simulink model "VCU_GearMgnt"  (R2023b)
settings: Solver=FixedStepDiscrete  StartTime=0.0  StopTime=10  FixedStep=0.01  RelTol=1e-3
undefined symbols (not defined in the file or in its folder): MOTOR_RPM_EN_GEAR, VEH_SPEED_EN_GEAR
libraries: simulink x24
settings Model: Creator=Administrator  LastModifiedBy=Administrator
settings OptimizationCC: DefaultParameterBehavior=Inlined  EnhancedBackFolding=on  PassReuseOutputArgsAs=Individual arguments  ZeroExternalMemoryAtStartup=off  ZeroInternalMemoryAtStartup=off  OptimizeBlockOrder=speed  DifferentSizesBufferReuse=on  OptimizationCustomize=off  EfficientTunableParamExpr=on
settings DebuggingCC: ParameterTunabilityLossMsg=error
settings HardwareCC: ProdBitPerPointer=32  ProdBitPerSizeT=32  ProdBitPerPtrDiffT=32  ProdLargestAtomicInteger=Long  ProdLargestAtomicFloat=Double  ProdWordSize=32  ProdHWDeviceType=ARM Compatible->ARM Cortex-M
settings SFSimCC: MATLABDynamicMemAlloc=off
settings RTWCC: Description=Embedded Coder  SystemTargetFile=ert.tlc  GenCodeOnly=on  TemplateMakefile=ert_default_tmf  GenerateReport=on  IncludeHyperlinkInReport=on  LaunchReport=on  GenerateTraceInfo=on  GenerateTraceReport=on  GenerateCodeReplacementReport=on
settings CodeAppCC: ForceParamTrailComments=on  IgnoreCustomStorageClasses=off  OperatorAnnotations=on  SimulinkDataObjDesc=on  SFDataObjDesc=on  InsertBlockDesc=on
settings ERTTargetCC: TargetLangStandard=C99 (ISO)  GenerateSampleERTMain=on  InlinedParameterPlacement=NonHierarchical  ERTCustomFileTemplate=example_file_process.tlc

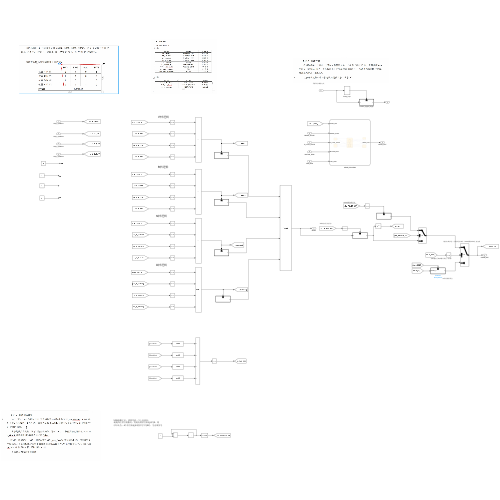
[thumbnail: Simulink's stored preview of the top-level diagram]
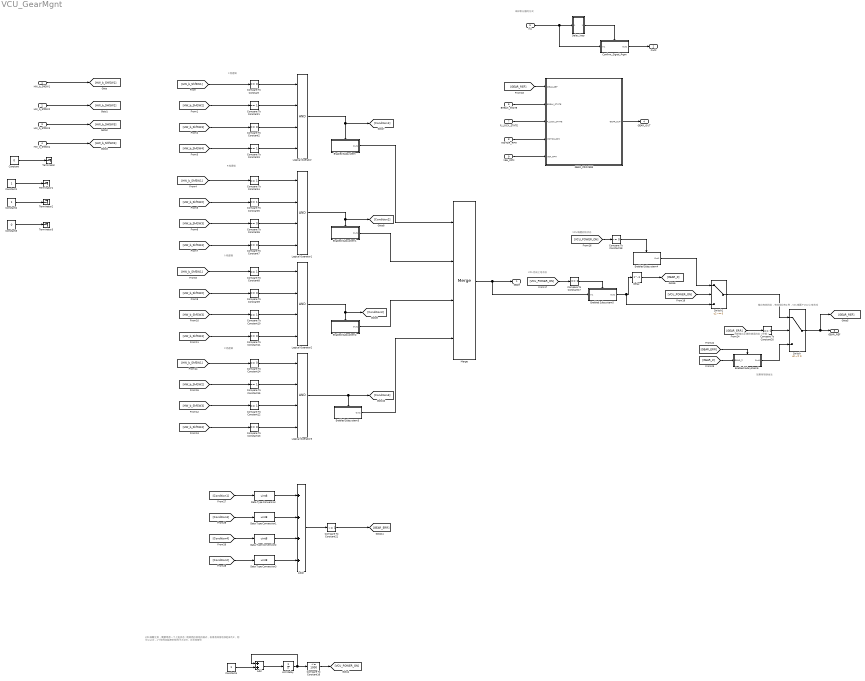
== system VCU_GearMgnt ==
  note: P档逻辑
  note: 输出有效挡位，有效挡位有2种，VCU唤醒+VCU上电完成
  note: 如果有错误发生
  note: VCU唤醒初始状态
  note: VCU唤醒之后，需要考虑一个上电状态;
      | 观测挡位信号的格式，发现有效信号加起来为2，则
      | 可以认为，4个信号加起来的信号不为2时，为无效信号
  note: 采样积分器的方式
  note: VCU完成上电状态
  note: 判断输出正确和错误挡位（仲裁）
  note: R档逻辑
  note: N档逻辑
  note: D档逻辑
  HW_b_ShfSW1 : Inport
  HW_b_ShfSW2 : Inport  Port=2
  HW_b_ShfSW3 : Inport  Port=3
  HW_b_ShfSW4 : Inport  Port=4
  In1 : Inport  Port=5
  BREAK_STATE : Inport  Port=6
  P_LOCK_STATE : Inport  Port=7
  MOTOR_RPM : Inport  Port=8
  VEH_RPM : Inport  Port=9
  Add : Sum
  Add2 : Sum  Inputs=++++
  Compare To Constant{,2,6..7,9,11,13..14,17,20} (10 alike) : simulink/Logic and Bit Operations/Compare To Constant  relop===  const=0  OutDataTypeStr=boolean
  Compare To Constant{1,3..5,8,10,12,15} (8 alike) : simulink/Logic and Bit Operations/Compare To Constant  relop===  const=1  OutDataTypeStr=boolean
  Compare To Constant16 : simulink/Logic and Bit Operations/Compare To Constant  relop=<=  const=1000  OutDataTypeStr=boolean
  Compare To Constant18 : simulink/Logic and Bit Operations/Compare To Constant  relop=~=  const=0  OutDataTypeStr=boolean
  Compare To Constant21 : simulink/Logic and Bit Operations/Compare To Constant  relop=~=  const=1  OutDataTypeStr=boolean
  Confirm_Signal_Prgm : Subsystem  TreatAsAtomicUnit=on
  Constant : Constant  Value=0
  Constant1 : Constant
  Constant2 : Constant
  Constant3 : Constant  Value=0
  Constant4 : Constant
  Data Type Conversion{,1..3} (4 alike) : DataTypeConversion  OutDataTypeStr=uint8  SaturateOnIntegerOverflow=off  RndMeth=Floor
  Delay : Delay  DelayLength=1  InputProcessing=Columns as channels (frame based)
  Delay_loop : Subsystem
  Enabled Subsystem : Subsystem  TreatAsAtomicUnit=on
  Enabled Subsystem1 : Subsystem  TreatAsAtomicUnit=on
  Enabled Subsystem2 : Subsystem  TreatAsAtomicUnit=on
  Enabled Subsystem3 : Subsystem  TreatAsAtomicUnit=on
  Enabled Subsystem4 : Subsystem  TreatAsAtomicUnit=on
  Enabled Subsystem5 : Subsystem  TreatAsAtomicUnit=on
  Enabled Subsystem6 : Subsystem  TreatAsAtomicUnit=on
  GEAR_PROCESS : Stateflow chart  TreatAsAtomicUnit=on
  Logical Operator{,1..3} (4 alike) : Logic  Inputs=4  AllPortsSameDT=off  OutDataTypeStr=boolean
  Merge : Merge  Inputs=4
  Switch : Switch  Criteria=u2 ~= 0  SaturateOnIntegerOverflow=off  InputSameDT=off
  Switch1 : Switch  Criteria=u2 ~= 0  SaturateOnIntegerOverflow=off  InputSameDT=off
  Terminator{,1..3} (4 alike) : Terminator
  Unit Delay : UnitDelay  SampleTime=-1  HasFrameUpgradeWarning=on
  GEAR : Outport
  Out2 : Outport  Port=2
  GEAR_REF : Outport  Port=3
  GEAR_OUT : Outport  Port=4
  wires:
  [HW_b_ShfSW1] -> Compare To Constant/1
  [HW_b_ShfSW2] -> Compare To Constant1/1
  [HW_b_ShfSW3] -> Compare To Constant2/1
  [HW_b_ShfSW4] -> Compare To Constant3/1
  Compare To Constant/1 -> Logical Operator/1
  Compare To Constant1/1 -> Logical Operator/2
  Compare To Constant2/1 -> Logical Operator/3
  Compare To Constant3/1 -> Logical Operator/4
  Compare To Constant7/1 -> Logical Operator1/4
  Compare To Constant6/1 -> Logical Operator1/3
  Compare To Constant5/1 -> Logical Operator1/2
  Compare To Constant4/1 -> Logical Operator1/1
  [HW_b_ShfSW4] -> Compare To Constant7/1
  [HW_b_ShfSW3] -> Compare To Constant6/1
  [HW_b_ShfSW2] -> Compare To Constant5/1
  [HW_b_ShfSW1] -> Compare To Constant4/1
  [HW_b_ShfSW1] -> Compare To Constant8/1
  [HW_b_ShfSW2] -> Compare To Constant9/1
  [HW_b_ShfSW3] -> Compare To Constant10/1
  [HW_b_ShfSW4] -> Compare To Constant11/1
  Compare To Constant8/1 -> Logical Operator2/1
  Compare To Constant9/1 -> Logical Operator2/2
  Compare To Constant10/1 -> Logical Operator2/3
  Compare To Constant11/1 -> Logical Operator2/4
  Compare To Constant13/1 -> Logical Operator3/4
  Compare To Constant12/1 -> Logical Operator3/3
  Compare To Constant15/1 -> Logical Operator3/2
  Compare To Constant14/1 -> Logical Operator3/1
  [HW_b_ShfSW4] -> Compare To Constant13/1
  [HW_b_ShfSW3] -> Compare To Constant12/1
  [HW_b_ShfSW2] -> Compare To Constant15/1
  [HW_b_ShfSW1] -> Compare To Constant14/1
  Logical Operator/1 -> [Condition1], Enabled Subsystem/Enable
  Logical Operator1/1 -> Enabled Subsystem1/Enable, [Condition2]
  Logical Operator2/1 -> [Condition3], Enabled Subsystem2/Enable
  Logical Operator3/1 -> Enabled Subsystem3/Enable, [Condition4]
  Enabled Subsystem/1(Out1) -> Merge/1
  Enabled Subsystem1/1(Out1) -> Merge/2
  Enabled Subsystem2/1(Out1) -> Merge/3
  Enabled Subsystem3/1(Out1) -> Merge/4
  Merge/1 -> Enabled Subsystem5/1(In1), GEAR/1
  HW_b_ShfSW1/1 -> [HW_b_ShfSW1]
  HW_b_ShfSW2/1 -> [HW_b_ShfSW2]
  HW_b_ShfSW3/1 -> [HW_b_ShfSW3]
  HW_b_ShfSW4/1 -> [HW_b_ShfSW4]
  Constant/1 -> Terminator/1
  Constant1/1 -> Terminator1/1
  Constant2/1 -> Terminator2/1
  Constant3/1 -> Terminator3/1
  In1/1 -> Confirm_Signal_Prgm/1(In1), Delay_loop/1(In1)
  Delay_loop/1(Out2) -> Confirm_Signal_Prgm/Enable
  Confirm_Signal_Prgm/1(Out1) -> Out2/1
  Constant4/1 -> Add/2
  Add/1 -> Unit Delay/1
  Unit Delay/1 -> Add/1, Compare To Constant16/1
  Compare To Constant16/1 -> [VCU_POWER_ON]
  [VCU_POWER_ON] -> Compare To Constant18/1
  [VCU_POWER_ON] -> Compare To Constant17/1
  Compare To Constant17/1 -> Enabled Subsystem5/Enable
  Compare To Constant18/1 -> Enabled Subsystem4/Enable
  Enabled Subsystem5/1(Out1) -> Delay/1, Switch1/3
  Delay/1 -> [GEAR_Z]
  [GEAR_ERR] -> Enabled Subsystem6/Enable
  [GEAR_Z] -> Enabled Subsystem6/1(GEAR_Z)
  [GEAR_ERR] -> Compare To Constant20/1
  Compare To Constant20/1 -> Switch/2
  Enabled Subsystem4/1(Out1) -> Switch1/1
  [VCU_POWER_ON] -> Switch1/2
  Switch1/1 -> Switch/1
  Enabled Subsystem6/1(Out1) -> Switch/3
  Switch/1 -> GEAR_REF/1, [GEAR_REF]
  [Condition1] -> Data Type Conversion/1
  [Condition3] -> Data Type Conversion1/1
  [Condition4] -> Data Type Conversion2/1
  [Condition2] -> Data Type Conversion3/1
  Add2/1 -> Compare To Constant21/1
  Compare To Constant21/1 -> [GEAR_ERR]
  Data Type Conversion/1 -> Add2/1
  Data Type Conversion1/1 -> Add2/2
  Data Type Conversion2/1 -> Add2/3
  Data Type Conversion3/1 -> Add2/4
  [GEAR_REF] -> GEAR_PROCESS/1(GEAR_REF)
  BREAK_STATE/1 -> GEAR_PROCESS/2(BREAK_STATE)
  P_LOCK_STATE/1 -> GEAR_PROCESS/3(P_LOCK_STATE)
  MOTOR_RPM/1 -> GEAR_PROCESS/4(MOTOR_RPM)
  VEH_RPM/1 -> GEAR_PROCESS/5(VEH_RPM)
  GEAR_PROCESS/1(GEAR_OUT) -> GEAR_OUT/1

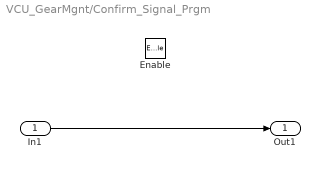
== system VCU_GearMgnt/Confirm_Signal_Prgm ==
  In1 : Inport
  Enable : EnablePort
  Out1 : Outport
  wires:
  In1/1 -> Out1/1

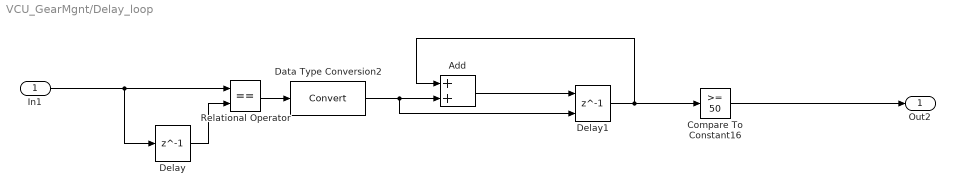
== system VCU_GearMgnt/Delay_loop ==
  In1 : Inport
  Add : Sum
  Compare To Constant16 : simulink/Logic and Bit Operations/Compare To Constant  relop=>=  const=50  OutDataTypeStr=boolean
  Data Type Conversion2 : DataTypeConversion  SaturateOnIntegerOverflow=off  RndMeth=Floor
  Delay : Delay  DelayLength=1  InputProcessing=Columns as channels (frame based)
  Delay1 : Delay  DelayLength=1  ExternalReset=Falling  InputProcessing=Columns as channels (frame based)
      settings: InputPortMap=u0,r5
  Relational Operator : RelationalOperator  Operator===  OutDataTypeStr=boolean  RndMeth=Simplest  InputSameDT=off
  Out2 : Outport
  wires:
  Delay/1 -> Relational Operator/2
  Add/1 -> Delay1/1
  Delay1/1 -> Compare To Constant16/1, Add/1
  Compare To Constant16/1 -> Out2/1
  Relational Operator/1 -> Data Type Conversion2/1
  In1/1 -> Delay/1, Relational Operator/1
  Data Type Conversion2/1 -> Delay1/2, Add/2

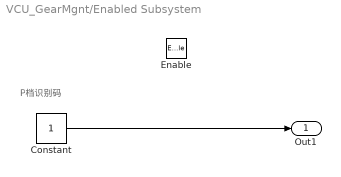
== system VCU_GearMgnt/Enabled Subsystem ==
  note: P档识别码
  Enable : EnablePort
  Constant : Constant
  Out1 : Outport
  wires:
  Constant/1 -> Out1/1

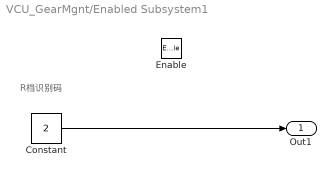
== system VCU_GearMgnt/Enabled Subsystem1 ==
  note: R档识别码
  Enable : EnablePort
  Constant : Constant  Value=2
  Out1 : Outport
  wires:
  Constant/1 -> Out1/1

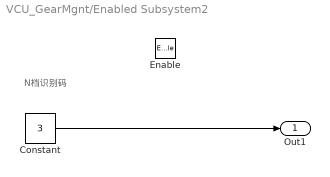
== system VCU_GearMgnt/Enabled Subsystem2 ==
  note: N档识别码
  Enable : EnablePort
  Constant : Constant  Value=3
  Out1 : Outport
  wires:
  Constant/1 -> Out1/1

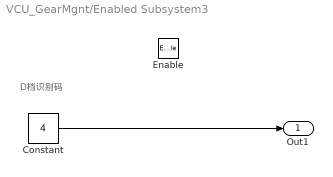
== system VCU_GearMgnt/Enabled Subsystem3 ==
  note: D档识别码
  Enable : EnablePort
  Constant : Constant  Value=4
  Out1 : Outport
  wires:
  Constant/1 -> Out1/1

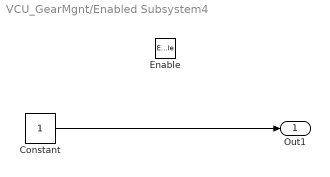
== system VCU_GearMgnt/Enabled Subsystem4 ==
  Enable : EnablePort
  Constant : Constant
  Out1 : Outport
  wires:
  Constant/1 -> Out1/1

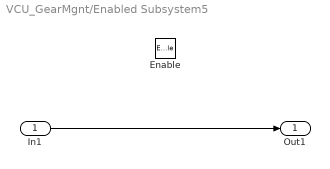
== system VCU_GearMgnt/Enabled Subsystem5 ==
  In1 : Inport
  Enable : EnablePort
  Out1 : Outport
  wires:
  In1/1 -> Out1/1

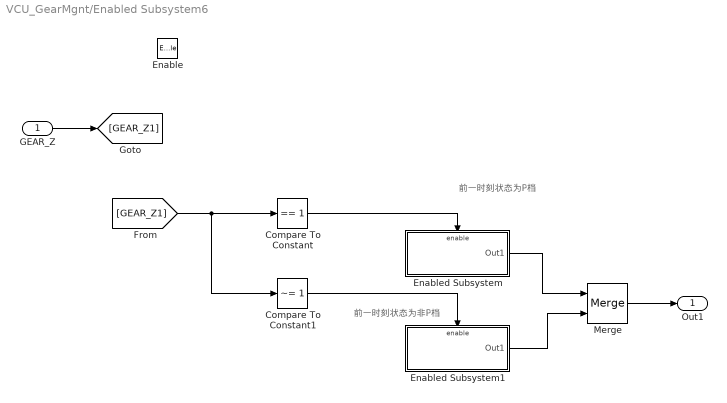
== system VCU_GearMgnt/Enabled Subsystem6 ==
  note: 前一时刻状态为P档
  note: 前一时刻状态为非P档
  GEAR_Z : Inport
  Enable : EnablePort
  Compare To Constant : simulink/Logic and Bit Operations/Compare To Constant  relop===  const=1  OutDataTypeStr=boolean
  Compare To Constant1 : simulink/Logic and Bit Operations/Compare To Constant  relop=~=  const=1  OutDataTypeStr=boolean
  Enabled Subsystem : Subsystem  TreatAsAtomicUnit=on
  Enabled Subsystem1 : Subsystem  TreatAsAtomicUnit=on
  Merge : Merge
  Out1 : Outport
  wires:
  GEAR_Z/1 -> [GEAR_Z1]
  [GEAR_Z1] -> Compare To Constant1/1, Compare To Constant/1
  Compare To Constant/1 -> Enabled Subsystem/Enable
  Compare To Constant1/1 -> Enabled Subsystem1/Enable
  Enabled Subsystem/1(Out1) -> Merge/1
  Enabled Subsystem1/1(Out1) -> Merge/2
  Merge/1 -> Out1/1

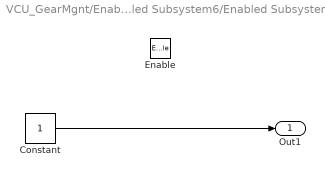
== system VCU_GearMgnt/Enabled Subsystem6/Enabled Subsystem ==
  Enable : EnablePort
  Constant : Constant  OutDataTypeStr=uint8
  Out1 : Outport
  wires:
  Constant/1 -> Out1/1

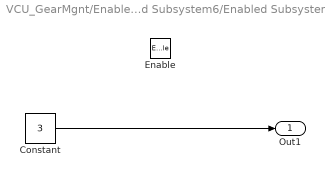
== system VCU_GearMgnt/Enabled Subsystem6/Enabled Subsystem1 ==
  Enable : EnablePort
  Constant : Constant  Value=3  OutDataTypeStr=uint8
  Out1 : Outport
  wires:
  Constant/1 -> Out1/1

== stateflow chart VCU_GearMgnt/GEAR_PROCESS ==
  state N_STATE
    en:
    GEAR_OUT = 3;
  state P_STATE
    en:
    GEAR_OUT = 1;
  state SHIFT_STATE
    state P_SHIFT
    state NP_SHIFT
    (default) -> P_SHIFT
    P_SHIFT -> NP_SHIFT [order 1] : [GEAR ~= 1]
    NP_SHIFT -> P_SHIFT [order 3] : [GEAR == 1]
  note: P2N
  note: N2P
  note: P2R
  note: R2P
  note: R2N
  note: D2P
  note: D2N
  state D_STATE
    en:
    GEAR_OUT = 4;
  note: P2D
  state R_STATE
    GEAR_OUT = 2;
  note: N2R
  note: D2R
  note: R2D
  (default) -> P_STATE
  P_STATE -> SHIFT_STATE : [GEAR_REF ~= 1]
  N_STATE -> SHIFT_STATE : [GEAR_REF ~= 3]
  P_SHIFT -> N_STATE [order 2] : [(GEAR_REF == 3) && (BREAK == 1) && (P_LOCK_STATE == 0)]
  NP_SHIFT -> N_STATE [order 4] : [GEAR_REF == 3]
  NP_SHIFT -> P_STATE [order 5] : [(GEAR == 1) && (VEH_RPM < VEH_SPEED_EN_GEAR)]
  P_SHIFT -> R_STATE [order 4] : [(GEAR_REF == 2) && (BREAK == 1)&&(MOTOR < MOTOR_RPM_EN_GEAR)&&...
      | (P_LOCK_STATE == 0)]
  P_SHIFT -> D_STATE [order 3] : [(GEAR_REF == 4) && (BREAK == 1)&&(MOTOR < MOTOR_RPM_EN_GEAR)&&...
      | (P_LOCK_STATE == 0)]
  D_STATE -> SHIFT_STATE : [GEAR_REF ~= 4]
  R_STATE -> SHIFT_STATE : [GEAR_REF ~= 2]
  NP_SHIFT -> R_STATE [order 2] : [(GEAR_REF == 2) && (MOTOR < MOTOR_RPM_EN_GEAR)]
  NP_SHIFT -> D_STATE [order 1] : [(GEAR_REF == 4) && (MOTOR < MOTOR_RPM_EN_GEAR)]
  data: GEAR_REF input; BREAK_STATE input; P_LOCK_STATE input; MOTOR_RPM input; VEH_RPM input; MOTOR_RPM_EN_GEAR parameter; VEH_SPEED_EN_GEAR parameter; GEAR_OUT output
